simulink model "fzinfer_example_r13"  (Simulink 5.0)
settings: Solver=ode45  StartTime=0.0  StopTime=4  FixedStep=.25  RelTol=1e-3
undefined symbols (not defined in the file): mfs, rls
libraries: simulink x1
settings Model: Creator=lbusoniu  LastModifiedBy=lbusoniu  ExtModeAutoUpdateStatusClock=off  RTWOptions="-aEnforceIntegerDowncast=1 -aFoldNonRolledExpr=1 -aInlineInvariantSignals=0 -aInlineParameters=0 -aLocalBlockOutputs=1 -aRollThreshold=5 -aZeroInternalMemoryAtStartup=1 -aZeroExternalMemoryAtStartup=1 -aInitFltsAndDblsToZero=1 -aGenerateReport=0 -aGenCodeOnly=0 -aRTWVerbose=1 -aIncludeHyperlinkInReport=0 -aLaunchReport=0 -aForceParamTrailComments=0 -aGenerateComments=1 -aIgnoreCustomStorageClasses=1 -aIncHierarchyInIds=0 -aMaxRTWIdLen=31 -aShowEliminatedStatements=0 -aPrefixModelToSubsysFcnNames=1 -aIncDataTypeInIds=0 -aInsertBlockDesc=0 -aSimulinkBlockComments=1 -aInlinedPrmAccess=\"Literals\"  -aSuppressErrorStatus=0 -aModelReferenceCompliant=1 -aSupportNonInlinedSFcns=1 -aSupportContinuousTime=1 -aSupportComplex=1 -aSupportNonFinite=1 -aSupportAbsoluteTime=1 -aTargetFcnLib=\"ansi_tfl_tmw.mat\" -aMultiInstanceERTCode=0 -aLogVarNameModifier=\"rt_\" -aIsPILTarget=0 -aCombineOutputUpdateFcns=0 -aGenerateASAP2=0 -aGenerateSampleERTMain=0 -aGenerateFullHeader=1 -aUtilityFuncGeneration=\"Auto\" -aIncludeFileDelimiter=\"Auto\" -aIncludeMdlTerminateFcn=1 -aPurelyIntegerCode=0 -aERTCustomFileBanners=0 -aRTWCAPIStates=0 -aRTWCAPIParams=0 -aRTWCAPISignals=0 -aMatFileLogging=1 -aGenFloatMathFcnCalls=\"ANSI_C\" -aExtModeMexFile=\"ext_comm\" -aExtModeTransport=0 -aExtModeStaticAllocSize=1000000 -aExtModeTesting=0 -aExtModeStaticAlloc=0 -aExtMode=0"

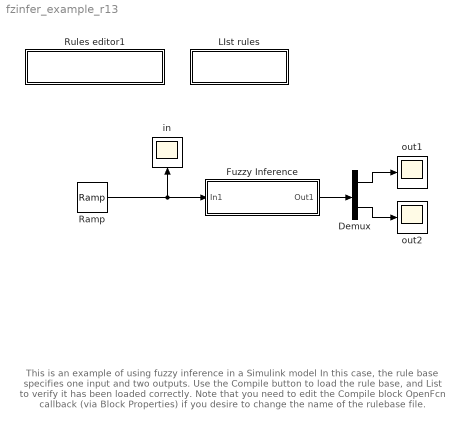
== system fzinfer_example_r13 ==
  note: This is an example of using fuzzy inference in a Simulink model
      |
      | In this case, the rule base specifies one input and two outputs.
      | Use the Compile button to load the rule base, and List to verify
      | it has been loaded correctly. Note that you need to edit the
      | Compile block OpenFcn callback (via Block Properties)
      | if you desire to change the name of the rulebase file.
  Demux : Demux  Outputs=2
  Fuzzy Inference : Subsystem  mask(Fuzzy inference block){rls=rls, mfs=mfs, def=[1 3]}
      mask prompts: rls "Rule matrix:"; mfs "Membership functions matrix:"; def "Default output:"
      mask help:
      | MIN-MAX inference with
      |  fuzzy means defuzzification
      mask Help: Fuzzy inference block can be used as a direct fuzzy controller or as a fuzzy supervisor. For details on dialog parameters see INFER.
      mask Display: disp('Fuzzy Inference')
  LIst rules : Subsystem  Orientation=down
      settings: OpenFcn=disp(rls2txt(rls, mfs, inputs, outputs, nlab, labels));
      mask Display: disp('List Fuzzy Rules')
  Ramp : simulink/Sources/Ramp  slope=1  start=0  X0=0
  Rules editor1 : Subsystem  Orientation=down
      settings: OpenFcn=eval(['[rls, mfs, inputs, outputs, nlab, labels] = txt2rls(''rulebase.rb'');']);
      mask Type: Rule-base editor
      mask Display: disp('Compile Rulebase')
  in : Scope
      settings: Orientation=up  TimeRange=4  YMin=0  YMax=4  SaveName=ScopeData2
  out1 : Scope
      settings: TimeRange=4  YMin=1  YMax=4
  out2 : Scope
      settings: TimeRange=4  YMin=1  YMax=3
  wires:
  Fuzzy Inference/1(Out1) -> Demux/1
  Demux/1 -> out1/1
  Demux/2 -> out2/1
  Ramp/1 -> Fuzzy Inference/1(In1), in/1

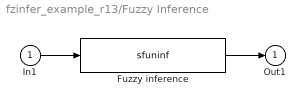
== system fzinfer_example_r13/Fuzzy Inference ==
  In1 : Inport
  Fuzzy inference : S-Function  FunctionName=sfuninf  Parameters=rls, mfs, def
  Out1 : Outport
  wires:
  In1/1 -> Fuzzy inference/1
  Fuzzy inference/1 -> Out1/1

== system fzinfer_example_r13/LIst rules ==

== system fzinfer_example_r13/Rules editor1 ==
